simulink model "Encoder"  (R2018b)
settings: Solver=FixedStepDiscrete  StartTime=0.0  StopTime=inf  FixedStep=0.005  RelTol=1e-3  EnableMultiTasking=on
libraries: arduinolib x2, dspswit3 x1, simulink x1
settings Model: SimulationMode=external  ExtModeTrigDuration=2  Creator=Yago  LastModifiedBy=Yago
settings OptimizationCC: EnhancedBackFolding=on  PassReuseOutputArgsAs=Individual arguments  MaxStackSize=64  OptimizeBlockOrder=speed  DifferentSizesBufferReuse=on  OptimizationCustomize=off
settings DebuggingCC: ParameterTunabilityLossMsg=error
settings HardwareCC: ProdBitPerInt=16  ProdBitPerPointer=16  ProdBitPerSizeT=16  ProdBitPerPtrDiffT=16  ProdLargestAtomicFloat=None  ProdWordSize=8  ProdHWDeviceType=Atmel->AVR
settings SFSimCC: MATLABDynamicMemAlloc=off
settings RTWCC: SystemTargetFile=ert.tlc  HardwareBoard=Arduino Uno  TemplateMakefile=ert_default_tmf  GenerateReport=on  Toolchain=Arduino AVR  BuildConfiguration=Faster Runs  IncludeHyperlinkInReport=on  LaunchReport=on  GenerateTraceInfo=on  GenerateTraceReport=on  GenerateTraceReportSl=on  GenerateTraceReportSf=on  GenerateTraceReportEml=on
settings CodeAppCC: ForceParamTrailComments=on  IgnoreCustomStorageClasses=off  OperatorAnnotations=on  SimulinkDataObjDesc=on  SFDataObjDesc=on  InsertBlockDesc=on
settings ERTTargetCC: SupportContinuousTime=on  SupportVariableSizeSignals=on

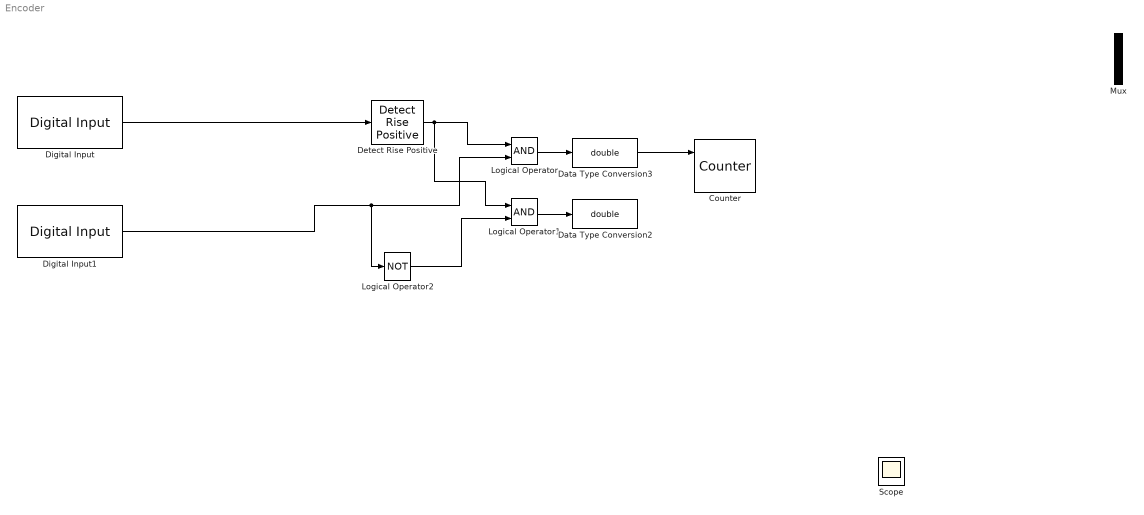
== system Encoder ==
  Counter : dspswit3/Counter  Direction=Up  CountEvent=Rising edge  CounterSize=32 bits  MaxCount=255  InitialCount=0  Output=Count  HitValue=32  ResetInput=on  SamplesPerFrame=1  Ts=1  CntDtype=double  HitDtype=Logical
  Data Type Conversion2 : DataTypeConversion  OutDataTypeStr=double
  Data Type Conversion3 : DataTypeConversion  OutDataTypeStr=double  LockScale=on
  Detect Rise Positive : simulink/Logic and Bit Operations/Detect Rise Positive  vinit=0  OutDataTypeStr=boolean
  Digital Input : arduinolib/Digital Input  pinNumber=3  sampleTime=0.005  blockPlatform=arduino
      settings: SourceProductName=Simulink Support Package for Arduino Hardware
  Digital Input1 : arduinolib/Digital Input  pinNumber=2  sampleTime=0.005  blockPlatform=arduino
      settings: SourceProductName=Simulink Support Package for Arduino Hardware
  Logical Operator : Logic  AllPortsSameDT=off  OutDataTypeStr=boolean
  Logical Operator1 : Logic  AllPortsSameDT=off  OutDataTypeStr=boolean
  Logical Operator2 : Logic  Operator=NOT  AllPortsSameDT=off  OutDataTypeStr=boolean
  Mux : Mux
  Scope : Scope
  wires:
  Detect Rise Positive/1 -> Logical Operator1/1, Logical Operator/1
  Digital Input1/1 -> Logical Operator/2, Logical Operator2/1
  Logical Operator2/1 -> Logical Operator1/2
  Logical Operator1/1 -> Data Type Conversion2/1
  Logical Operator/1 -> Data Type Conversion3/1
  Digital Input/1 -> Detect Rise Positive/1
  Data Type Conversion3/1 -> Counter/1
